simulink model "Observer"  (R2017b)
settings: Solver=VariableStepAuto  StartTime=0.0  StopTime=2  FixedStep=1e-5  RelTol=1e-3  EnableMultiTasking=on
undefined symbols (not defined in the file): DiscIntNeverNeededParam, J, K, Kf, L, PID_Ki, PID_Kp, Pos_Kp, R, Spd_Ki, Spd_Kp, SPD_LIN_KI, SPD_LIN_KP, SPD_SM_K1, SPD_SM_K2
libraries: simulink_extras x2
settings Model: Creator=uids8840  LastModifiedBy=uids8840
settings SolverCC: AlgebraicLoopSolver=LineSearch
settings DataIOCC: LimitDataPoints=on  SaveFormat=Array  SaveOutput=off  SignalLogging=off  DSMLogging=off  SaveTime=off
settings OptimizationCC: BooleanDataType=off  LifeSpan=inf
settings DebuggingCC: UnderspecifiedInitializationDetection=Classic  MergeDetectMultiDrivingBlocksExec=none  SolverPrmCheckMsg=warning  MultiTaskRateTransMsg=warning  SFUnexpectedBacktrackingDiag=warning  SFNoUnconditionalDefaultTransitionDiag=warning  SFExecutionAtInitializationDiag=none
settings HardwareCC: ProdBitPerPointer=32  ProdBitPerSizeT=32  ProdBitPerPtrDiffT=32  ProdLargestAtomicFloat=None  ProdIntDivRoundTo=Undefined  ProdEndianess=Unspecified  ProdWordSize=32  ProdHWDeviceType=32-bit Generic
settings ModelReferenceCC: UpdateModelReferenceTargets=IfOutOfDate  ModelReferenceNumInstancesAllowed=Single  PropagateSignalLabelsOutOfModel=off
settings SFSimCC: SFSimEcho=off  SimCtrlC=off  SimIntegrity=off
settings CodeAppCC: StateflowObjectComments=on
settings GRTTargetCC: TargetLangStandard=C89/C90 (ANSI)  GeneratePreprocessorConditionals=Disable all
settings ConfigComp: CovMetricSettings=dw  CovHtmlReporting=on  CovSaveCumulativeToWorkspaceVar=on  CovSaveSingleToWorkspaceVar=on  CovExternalEMLEnable=off

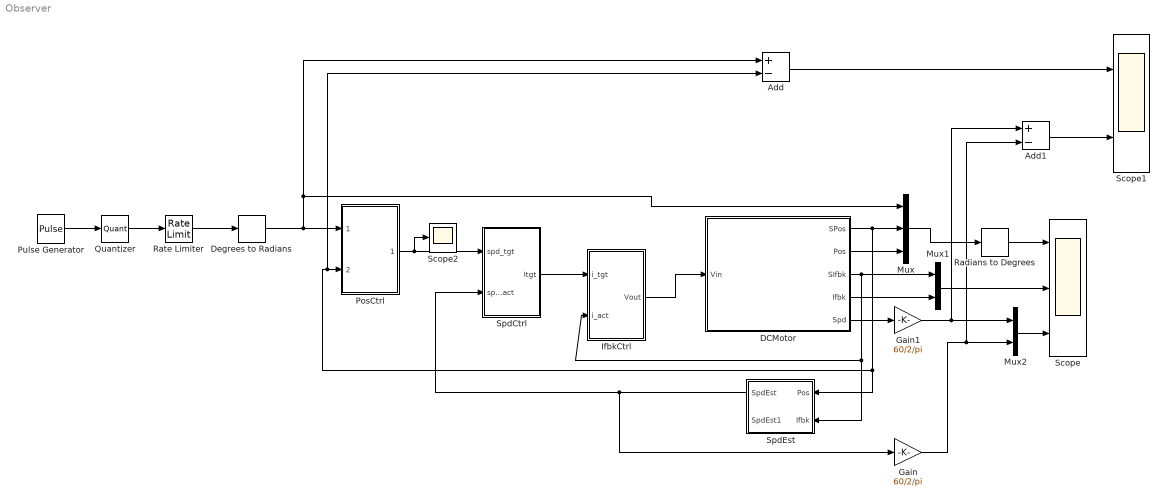
== system Observer ==
  Add : Sum  Inputs=+-
  Add1 : Sum  Inputs=+-
  DCMotor : Subsystem
  Degrees to Radians : simulink_extras/Transformations/Degrees to Radians
  Gain : Gain  Gain=60/2/pi
  Gain1 : Gain  Gain=60/2/pi
  IfbkCtrl : Subsystem  TreatAsAtomicUnit=on  SystemSampleTime=1e-4
  Mux : Mux  Inputs=3
  Mux1 : Mux  Inputs=2
  Mux2 : Mux  Inputs=2
  PosCtrl : Subsystem  TreatAsAtomicUnit=on  SystemSampleTime=1e-3
  Pulse Generator : DiscretePulseGenerator  PulseType=Time based  Amplitude=100  Period=0.5  PulseWidth=50
  Quantizer : Quantizer  QuantizationInterval=2*pi/400
  Radians to Degrees : simulink_extras/Transformations/Radians to Degrees
  Rate Limiter : RateLimiter  RisingSlewLimit=1000  FallingSlewLimit=-1000  SampleTimeMode=inherited
  Scope : Scope  NumInputPorts=3
  Scope1 : Scope  NumInputPorts=2
  Scope2 : Scope
  SpdCtrl : Subsystem  TreatAsAtomicUnit=on  SystemSampleTime=1e-3
  SpdEst : Subsystem  TreatAsAtomicUnit=on  SystemSampleTime=1e-4
  wires:
  DCMotor/1(SPos) -> Mux/2, Add/2, PosCtrl/2(pos_act), SpdEst/1(Pos)
  DCMotor/3(SIfbk) -> IfbkCtrl/2(i_act), SpdEst/2(Ifbk), Mux1/1
  Mux/1 -> Radians to Degrees/1
  DCMotor/4(Ifbk) -> Mux1/2
  Mux1/1 -> Scope/2
  SpdCtrl/1(Itgt) -> IfbkCtrl/1(i_tgt)
  SpdEst/1(SpdEst) -> Gain/1, SpdCtrl/2(spd_act)
  PosCtrl/1(spdtgt) -> Scope2/1, SpdCtrl/1(spd_tgt)
  Degrees to Radians/1 -> Mux/1, Add/1, PosCtrl/1(pos_tgt)
  DCMotor/2(Pos) -> Mux/3
  IfbkCtrl/1(Vout) -> DCMotor/1(Vin)
  Radians to Degrees/1 -> Scope/1
  Quantizer/1 -> Rate Limiter/1
  Pulse Generator/1 -> Quantizer/1
  DCMotor/5(Spd) -> Gain1/1
  Mux2/1 -> Scope/3
  Gain/1 -> Add1/2, Mux2/2
  Add/1 -> Scope1/1
  Add1/1 -> Scope1/2
  Gain1/1 -> Add1/1, Mux2/1
  Rate Limiter/1 -> Degrees to Radians/1

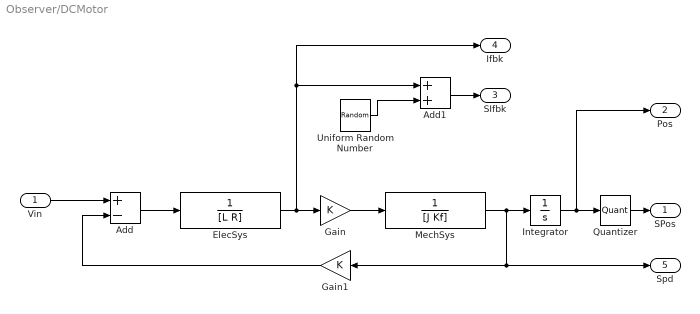
== system Observer/DCMotor ==
  Vin : Inport
  Add : Sum  Inputs=+-
  Add1 : Sum
  ElecSys : TransferFcn  Denominator=[L R]
  Gain : Gain  Gain=K
  Gain1 : Gain  Gain=K
  Integrator : Integrator
  MechSys : TransferFcn  Denominator=[J Kf]
  Quantizer : Quantizer  QuantizationInterval=2*pi/400
  Uniform Random Number : UniformRandomNumber  Minimum=-10e-3  Maximum=10e-3  SampleTime=1e-5
  SPos : Outport
  Pos : Outport  Port=2
  SIfbk : Outport  Port=3
  Ifbk : Outport  Port=4
  Spd : Outport  Port=5
  wires:
  Add/1 -> ElecSys/1
  ElecSys/1 -> Gain/1, Add1/1, Ifbk/1
  Gain/1 -> MechSys/1
  Vin/1 -> Add/1
  Quantizer/1 -> SPos/1
  MechSys/1 -> Integrator/1, Gain1/1, Spd/1
  Integrator/1 -> Pos/1, Quantizer/1
  Add1/1 -> SIfbk/1
  Uniform Random Number/1 -> Add1/2
  Gain1/1 -> Add/2

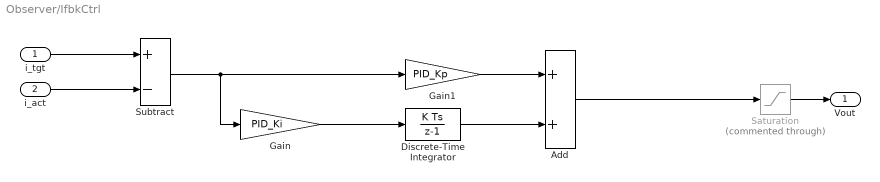
== system Observer/IfbkCtrl ==
  i_tgt : Inport
  i_act : Inport  Port=2
  Add : Sum
  Discrete-Time Integrator : DiscreteIntegrator  gainval=1  InitialConditionSetting=State (most efficient)  SampleTime=-1  OutDataTypeStr=Inherit: Inherit via back propagation  UpperSaturationLimit=100  LowerSaturationLimit=-100  ICPrevOutput=DiscIntNeverNeededParam  ICPrevScaledInput=DiscIntNeverNeededParam
  Gain : Gain  Gain=PID_Ki  ParamDataTypeStr=Inherit: Inherit from 'Gain'  OutDataTypeStr=Inherit: Inherit via back propagation
  Gain1 : Gain  Gain=PID_Kp  ParamDataTypeStr=Inherit: Inherit from 'Gain'  OutDataTypeStr=Inherit: Inherit via back propagation
  Saturation : Saturate  Commented=through  UpperLimit=12  LowerLimit=-12
  Subtract : Sum  Inputs=+-
  Vout : Outport
  wires:
  Saturation/1 -> Vout/1
  i_act/1 -> Subtract/2
  Gain1/1 -> Add/1
  Gain/1 -> Discrete-Time Integrator/1
  Subtract/1 -> Gain1/1, Gain/1
  Add/1 -> Saturation/1
  i_tgt/1 -> Subtract/1
  Discrete-Time Integrator/1 -> Add/2

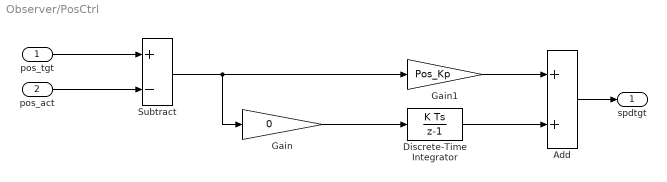
== system Observer/PosCtrl ==
  pos_tgt : Inport
  pos_act : Inport  Port=2
  Add : Sum
  Discrete-Time Integrator : DiscreteIntegrator  gainval=1  InitialConditionSetting=State (most efficient)  SampleTime=-1  OutDataTypeStr=Inherit: Inherit via back propagation  UpperSaturationLimit=100  LowerSaturationLimit=-100  ICPrevOutput=DiscIntNeverNeededParam  ICPrevScaledInput=DiscIntNeverNeededParam
  Gain : Gain  Gain=0  ParamDataTypeStr=Inherit: Inherit from 'Gain'  OutDataTypeStr=Inherit: Inherit via back propagation
  Gain1 : Gain  Gain=Pos_Kp  ParamDataTypeStr=Inherit: Inherit from 'Gain'  OutDataTypeStr=Inherit: Inherit via back propagation
  Subtract : Sum  Inputs=+-
  spdtgt : Outport
  wires:
  Add/1 -> spdtgt/1
  pos_act/1 -> Subtract/2
  Gain1/1 -> Add/1
  Gain/1 -> Discrete-Time Integrator/1
  Subtract/1 -> Gain1/1, Gain/1
  pos_tgt/1 -> Subtract/1
  Discrete-Time Integrator/1 -> Add/2

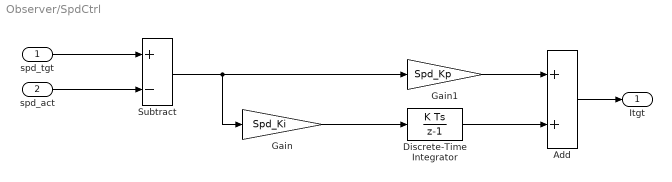
== system Observer/SpdCtrl ==
  spd_tgt : Inport
  spd_act : Inport  Port=2
  Add : Sum
  Discrete-Time Integrator : DiscreteIntegrator  gainval=1  InitialConditionSetting=State (most efficient)  SampleTime=-1  OutDataTypeStr=Inherit: Inherit via back propagation  UpperSaturationLimit=100  LowerSaturationLimit=-100  ICPrevOutput=DiscIntNeverNeededParam  ICPrevScaledInput=DiscIntNeverNeededParam
  Gain : Gain  Gain=Spd_Ki  ParamDataTypeStr=Inherit: Inherit from 'Gain'  OutDataTypeStr=Inherit: Inherit via back propagation
  Gain1 : Gain  Gain=Spd_Kp  ParamDataTypeStr=Inherit: Inherit from 'Gain'  OutDataTypeStr=Inherit: Inherit via back propagation
  Subtract : Sum  Inputs=+-
  Itgt : Outport
  wires:
  Discrete-Time Integrator/1 -> Add/2
  spd_tgt/1 -> Subtract/1
  Subtract/1 -> Gain/1, Gain1/1
  Gain/1 -> Discrete-Time Integrator/1
  Gain1/1 -> Add/1
  spd_act/1 -> Subtract/2
  Add/1 -> Itgt/1

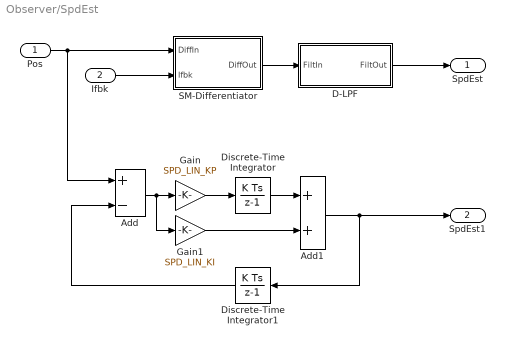
== system Observer/SpdEst ==
  Pos : Inport
  Ifbk : Inport  Port=2
  Add : Sum  Inputs=+-
  Add1 : Sum
  D-LPF : Subsystem
  Discrete-Time Integrator : DiscreteIntegrator  InitialConditionSetting=State (most efficient)  SampleTime=-1  ICPrevOutput=DiscIntNeverNeededParam  ICPrevScaledInput=DiscIntNeverNeededParam
  Discrete-Time Integrator1 : DiscreteIntegrator  InitialConditionSetting=State (most efficient)  SampleTime=-1  ICPrevOutput=DiscIntNeverNeededParam  ICPrevScaledInput=DiscIntNeverNeededParam
  Gain : Gain  Gain=SPD_LIN_KP
  Gain1 : Gain  Gain=SPD_LIN_KI
  SM-Differentiator : Subsystem
  SpdEst : Outport
  SpdEst1 : Outport  Port=2
  wires:
  Pos/1 -> Add/1, SM-Differentiator/1(DiffIn)
  SM-Differentiator/1(DiffOut) -> D-LPF/1(FiltIn)
  Add/1 -> Gain1/1, Gain/1
  Gain/1 -> Discrete-Time Integrator/1
  Discrete-Time Integrator/1 -> Add1/1
  Gain1/1 -> Add1/2
  Add1/1 -> SpdEst1/1, Discrete-Time Integrator1/1
  Discrete-Time Integrator1/1 -> Add/2
  D-LPF/1(FiltOut) -> SpdEst/1
  Ifbk/1 -> SM-Differentiator/2(Ifbk)

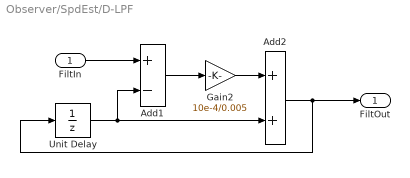
== system Observer/SpdEst/D-LPF ==
  FiltIn : Inport
  Add1 : Sum  Inputs=+-
  Add2 : Sum
  Gain2 : Gain  Gain=10e-4/0.005
  Unit Delay : UnitDelay  SampleTime=-1
  FiltOut : Outport
  wires:
  Add1/1 -> Gain2/1
  Gain2/1 -> Add2/1
  Unit Delay/1 -> Add1/2, Add2/2
  Add2/1 -> FiltOut/1, Unit Delay/1
  FiltIn/1 -> Add1/1

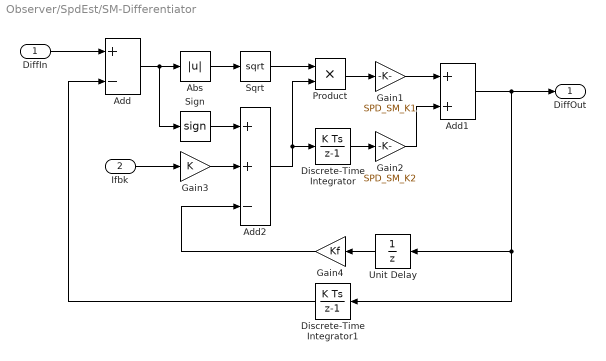
== system Observer/SpdEst/SM-Differentiator ==
  DiffIn : Inport
  Ifbk : Inport  Port=2
  Abs : Abs
  Add : Sum  Inputs=+-
  Add1 : Sum
  Add2 : Sum  Inputs=++-
  Discrete-Time Integrator : DiscreteIntegrator  InitialConditionSetting=State (most efficient)  SampleTime=-1  ICPrevOutput=DiscIntNeverNeededParam  ICPrevScaledInput=DiscIntNeverNeededParam
  Discrete-Time Integrator1 : DiscreteIntegrator  InitialConditionSetting=State (most efficient)  SampleTime=-1  ICPrevOutput=DiscIntNeverNeededParam  ICPrevScaledInput=DiscIntNeverNeededParam
  Gain1 : Gain  Gain=SPD_SM_K1
  Gain2 : Gain  Gain=SPD_SM_K2
  Gain3 : Gain  Gain=K
  Gain4 : Gain  Gain=Kf
  Product : Product
  Sign : Signum
  Sqrt : Sqrt  SaturateOnIntegerOverflow=on
  Unit Delay : UnitDelay  SampleTime=-1
  DiffOut : Outport
  wires:
  Add/1 -> Sign/1, Abs/1
  Gain2/1 -> Add1/2
  Product/1 -> Gain1/1
  Discrete-Time Integrator/1 -> Gain2/1
  Add1/1 -> DiffOut/1, Unit Delay/1, Discrete-Time Integrator1/1
  Gain1/1 -> Add1/1
  Abs/1 -> Sqrt/1
  Add2/1 -> Product/2, Discrete-Time Integrator/1
  Discrete-Time Integrator1/1 -> Add/2
  Sqrt/1 -> Product/1
  DiffIn/1 -> Add/1
  Sign/1 -> Add2/1
  Gain3/1 -> Add2/2
  Ifbk/1 -> Gain3/1
  Gain4/1 -> Add2/3
  Unit Delay/1 -> Gain4/1
